simulink model "RandomResponseExperiment_SingleTank_2016a"  (R2016a)
settings: Solver=ode5  SolverMode=SingleTasking  StartTime=0.0  StopTime=1000  FixedStep=0.5  RelTol=1e-3
settings Model: Creator=HTH  LastModifiedBy=HTH
settings DebuggingCC: SFUnexpectedBacktrackingDiag=error  SFNoUnconditionalDefaultTransitionDiag=error
settings GRTTargetCC: TargetLangStandard=C99 (ISO)  GeneratePreprocessorConditionals=Use local settings
settings ConfigComp: CovMetricSettings=dwe  CovHtmlReporting=off  CovSaveCumulativeToWorkspaceVar=off  CovSaveSingleToWorkspaceVar=off  CovExternalEMLEnable=on

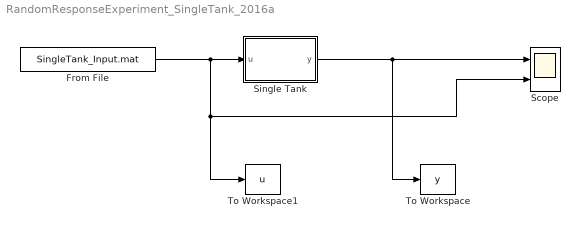
== system RandomResponseExperiment_SingleTank_2016a ==
  From File : FromFile  FileName=SingleTank_Input.mat
  Scope : Scope  NumInputPorts=2
  Single Tank : Subsystem  mask{K=60, A=200, b=1, C=0.8, g=981}
  To Workspace : ToWorkspace  VariableName=y  SampleTime=-1
  To Workspace1 : ToWorkspace  VariableName=u  SampleTime=-1
  wires:
  From File/1 -> Scope/2, To Workspace1/1, Single Tank/1(u)
  Single Tank/1(y) -> To Workspace/1, Scope/1

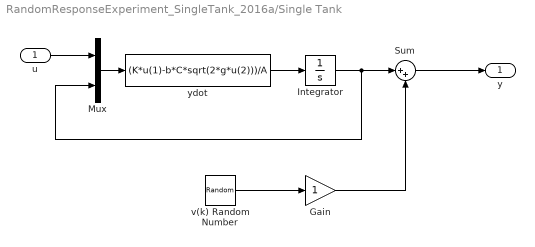
== system RandomResponseExperiment_SingleTank_2016a/Single Tank ==
  u : Inport
  Gain : Gain
  Integrator : Integrator  LimitOutput=on  UpperSaturationLimit=100  LowerSaturationLimit=0
  Mux : Mux  Inputs=2
  Sum : Sum  Inputs=|++
  v(k) Random Number : RandomNumber  Variance=0.1
  ydot : Fcn  Expr=(K*u(1)-b*C*sqrt(2*g*u(2)))/A
  y : Outport
  wires:
  Integrator/1 -> Mux/2, Sum/1
  ydot/1 -> Integrator/1
  Mux/1 -> ydot/1
  u/1 -> Mux/1
  Sum/1 -> y/1
  v(k) Random Number/1 -> Gain/1
  Gain/1 -> Sum/2
